simulink model "PFC"  (R2025a)
settings: Solver=VariableStepAuto  StartTime=0.0  StopTime=0.05  MaxStep=1e-9  RelTol=1e-3
libraries: spsDiodeLib x4, spsSeriesRLCBranchLib x2, spsACVoltageSourceLib x1, spsVoltageMeasurementLib x1, spspowerguiLib x1
settings Model: Creator=FCH  LastModifiedBy=FCH
settings DataIOCC: ReturnWorkspaceOutputs=off

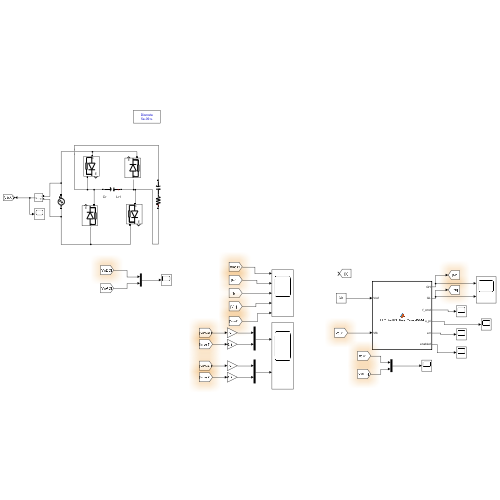
[thumbnail: Simulink's stored preview of the top-level diagram]
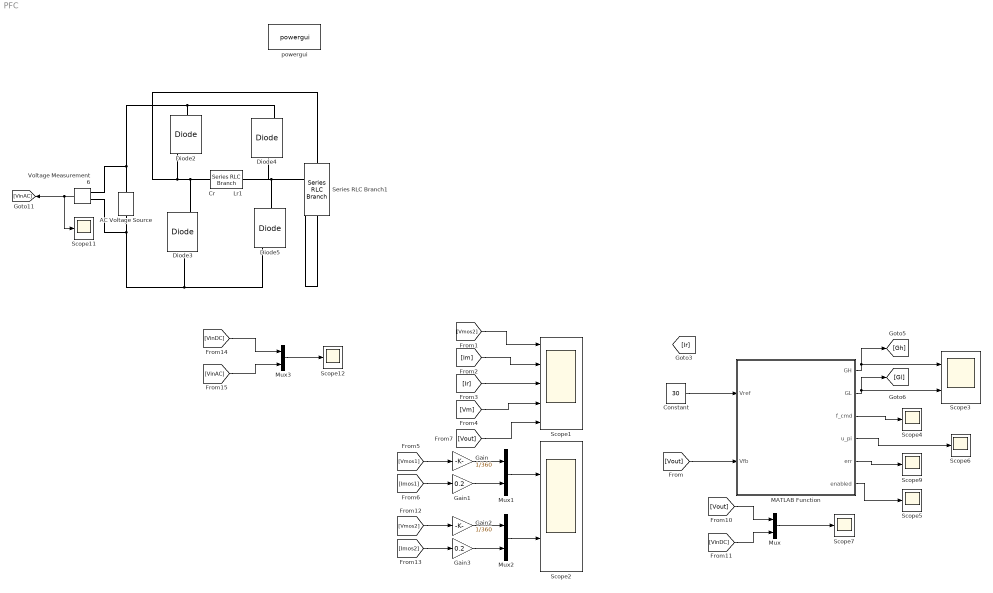
== system PFC ==
  AC Voltage Source : spsACVoltageSourceLib/AC Voltage Source  Amplitude=400  Phase=0  Frequency=50  SampleTime=0  Measurements=None  BusType=swing  Pref=10e3  Qref=0  Qmin=-inf  Qmax=+inf
  Constant : Constant  Value=30
  Cr           Lr1 : spsSeriesRLCBranchLib/Series RLC Branch  LConnTagsString=__new0  RConnTagsString=__new0  BranchType=C  Resistance=1000  Inductance=18e-6  SetiL0=off  InitialCurrent=0  Capacitance=1e-6  Setx0=off  InitialVoltage=0  Measurements=None
  Diode{2..5} (4 alike) : spsDiodeLib/Diode  Ron=0.001  Lon=0  Vf=0.8  IC=0  UseSnubber=0  Rs=500  Cs=250e-9  Measurements=on
  Gain : Gain  Gain=1/360
  Gain1 : Gain  Gain=0.2
  Gain2 : Gain  Gain=1/360
  Gain3 : Gain  Gain=0.2
  MATLAB Function : MATLAB Function  TreatAsAtomicUnit=on
  Mux{,1..3} (4 alike) : Mux  Inputs=2
  Scope1 : Scope  NumInputPorts=5
      settings: ActiveDisplayYMinimum=-50.08996079771358  ActiveDisplayYMaximum=450.08771732595056
  Scope{4..7,9,11..12} (7 alike) : Scope
      Scope11 settings: ActiveDisplayYMinimum=-499.86933273325383  ActiveDisplayYMaximum=498.82399459928456  DataLoggingVariableName=U_input1
      Scope12 settings: ActiveDisplayYMinimum=-62853.428585950089  ActiveDisplayYMaximum=-118.12720339930456  DataLoggingVariableName=ScopeData5
      Scope4 settings: ActiveDisplayYMinimum=222062.79129936235  ActiveDisplayYMaximum=225441.12510125362  DataLoggingVariableName=ScopeData4
      Scope5 settings: ActiveDisplayYMinimum=-0.12499999999999997  ActiveDisplayYMaximum=1.125  DataLoggingVariableName=ScopeData7
      Scope6 settings: ActiveDisplayYMinimum=-44.999999999999972  ActiveDisplayYMaximum=404.99999999999994  DataLoggingVariableName=ScopeData6
      Scope7 settings: ActiveDisplayYMinimum=-322.88834801894615  ActiveDisplayYMaximum=44.368039130053759  DataLoggingVariableName=ScopeData2
      Scope9 settings: ActiveDisplayYMinimum=-9.251113646286619  ActiveDisplayYMaximum=12.913805154194439  DataLoggingVariableName=ScopeData8
  Scope2 : Scope  NumInputPorts=2
      settings: ActiveDisplayYMinimum=-4.0516901529572973  ActiveDisplayYMaximum=20.70920117114095
  Scope3 : Scope  NumInputPorts=2
      settings: ActiveDisplayYMinimum=-0.12499999999999997  ActiveDisplayYMaximum=1.125  DataLoggingVariableName=ScopeData3
  Series RLC Branch1 : spsSeriesRLCBranchLib/Series RLC Branch  LConnTagsString=__new0  RConnTagsString=__new0  BranchType=RC  Resistance=0.01  Inductance=1e-3  SetiL0=off  InitialCurrent=0  Capacitance=1e-6  Setx0=off  InitialVoltage=0  Measurements=None
  Voltage Measurement6 : spsVoltageMeasurementLib/Voltage Measurement  PhasorSimulation=off  OutputType=Complex  PSBequivalent=0
  powergui : spspowerguiLib/powergui  Priority=1  SimulationMode=Discrete  SampleTime=1/(200e6)  frequency=60  Iterations=50  frequencyindice=0  Pbase=100e6  ErrMax=1e-4  UnitsV=kV  UnitsW=MW  buscounter=0  FunctionMessages=off  echomessages=off  EnableUseOfTLC=off  CurrentSourceSwitches=off  DisableSnubberDevices=off  DisableRonSwitches=off  DisableVfSwitches=off  DisplayEquations=off  AutomaticDiscreteSolvers=off  SolverType=Tustin/Backward Euler (TBE)  Interpol=off  ExternalGateDelay=off  methode=off  Ts=100  x0status=blocks  SPID=on  SwTol=0  HookPort=off  NonlinearTolerance=1e-4  nMaxIteration=100  ContinueOnMaxIteration=off  RestoreLinks=warning  ResistiveCurrentMeasurement=off  Frange=[0:2:500]  Ylog=off  Xlog=on  ShowGrid=off  save=off  variable=ZData  structure=0  ZoomFFT=off  StartTime=0.0  cycles=1  DisplayStyle=1  fundamental=60  FreqAxis=off  MaxFrequency=1000  frequencyindicesteady=1  RmsSteady=1  display=off
  wires:
  Constant/1 -> MATLAB Function/1(Vref)
  [Vout] -> MATLAB Function/2(Vfb)
  MATLAB Function/1(GH) -> [Gh], Scope3/1
  MATLAB Function/2(GL) -> [Gl], Scope3/2
  MATLAB Function/4(u_pi) -> Scope6/1
  MATLAB Function/3(f_cmd) -> Scope4/1
  MATLAB Function/5(err) -> Scope9/1
  [Vmos2] -> Scope1/1
  [Im] -> Scope1/2
  [Ir] -> Scope1/3
  [Vm] -> Scope1/4
  [Vout] -> Scope1/5
  Mux/1 -> Scope7/1
  [Vout] -> Mux/1
  [VinDC] -> Mux/2
  [Vmos1] -> Gain/1
  [Imos1] -> Gain1/1
  Mux1/1 -> Scope2/1
  [Vmos2] -> Gain2/1
  [Imos2] -> Gain3/1
  Mux2/1 -> Scope2/2
  Gain/1 -> Mux1/1
  Gain1/1 -> Mux1/2
  Gain2/1 -> Mux2/1
  Gain3/1 -> Mux2/2
  Voltage Measurement6/1 -> [VinAC], Scope11/1
  [VinDC] -> Mux3/1
  [VinAC] -> Mux3/2
  Mux3/1 -> Scope12/1
  MATLAB Function/6(enabled) -> Scope5/1
  connections:
  Cr           Lr1/LConn1 -- Diode4/LConn1 -- Series RLC Branch1/LConn1 -- Diode5/LConn1
  AC Voltage Source/RConn1 -- Diode4/RConn1 -- Diode2/LConn1 -- Voltage Measurement6/LConn2
  Diode5/RConn1 -- AC Voltage Source/LConn1 -- Voltage Measurement6/LConn1 -- Diode3/LConn1
  Diode2/RConn1 -- Series RLC Branch1/RConn1 -- Diode3/RConn1 -- Cr           Lr1/RConn1

== matlab function PFC/MATLAB Function ==
  data: Vref input; GH output; Vfb input; GL output; f_cmd output; u_pi output; err output; enabled output
function [GH, GL, f_cmd, u_pi, err, enabled] = LLC_VoltPI_Res_CompPWM(Vref, Vfb)
%#codegen
% LLC 变换器 PI 电压闭环 + 准谐振控制 + 互补 PWM 驱动（变频控制）
% 新增功能：准谐振控制消除9400Hz附近频率扰动
% 新增功能：0.02秒延时启动，0到0.02秒MOS管不导通
% 输入:
%   Vref  - 输出电压给定 (V)
%   Vfb   - 输出电压反馈 (V)
% 输出:
%   GH    - 高桥臂驱动（逻辑 0/1）
%   GL    - 低桥臂驱动（逻辑 0/1），与 GH 互补且带死区
%   f_cmd - 当前开关频率命令 (Hz)，便于观察
%   u_pi  - PI 控制器输出（归一化调节量，便于调试）
%   u_res - 准谐振控制器输出（便于调试）
%   u_total - 总控制输出（PI + 谐振）
%   err   - 误差值（便于调试）
%   enabled - 使能标志（0: 延时阶段，1: 正常运行）

% --- 控制周期（与 MATLAB Function 调用步长一致） ---
% Ts = 1/(270e3*20);          % 1 us 控制周期，例如 MCU 1 MHz ISR
Ts = 1/(2000e6);          % 0.5 ns 控制周期，用于高精度仿真
% Ts = 1/(1e6);             % 1 us 控制周期，MCU常见频率

% --- 启动延时参数 ---
startup_delay = 0.02/10;    % 启动延时 0.02 秒

% --- PI 参数（电压环）---
Kp = 0.00001;           % 比例系数
Ki = 50;                % 积分系数

% --- 准谐振控制器参数）---
Kr = 0.05;             % 谐振增益（需要根据实际调试）
f_res = 100;           % 谐振频率 (Hz) - 需要消除的扰动频率
omega_res = 2 * pi * f_res;  % 谐振角频率 (rad/s)

% 品质因数Q（影响带宽，Q越大带宽越窄，抑制越精确）
Q_res = 250000000;             % 品质因数

% --- LLC 开关频率范围 ---
f_min = 180e3;          % 最低频率 (Hz)
f_max = 270e3;          % 最高频率 (Hz)

% --- 死区时间 ---
t_dead = 186e-9;        % 200 ns 死区，根据驱动/器件调整

% --- 积分项限幅，防止积分饱和 ---
ui_max = 0.5;
ui_min = -0.5;

% --- 谐振控制器输出限幅 ---
u_res_max = 0.3;        % 谐振输出最大限幅
u_res_min = -0.3;       % 谐振输出最小限幅

% --- 总输出限幅 ---
u_total_max = 1.0;      % 总输出最大限幅
u_total_min = -1.0;     % 总输出最小限幅

%% ========= 持久变量（只初始化一次） =========
persistent ui t_half leg dead_t

% 准谐振控制器持久变量
persistent u_res_prev1 u_res_prev2  % 准谐振输出历史
persistent err_prev1 err_prev2      % 误差历史

% 离散化系数（只计算一次）
persistent b0_res b1_res b2_res a1_res a2_res

% 启动延时计时器
persistent startup_timer
persistent enable_flag

% 初始化
if isempty(ui)
    ui      = 0;        % PI 积分项
    t_half  = 0;        % 半周期计时
    leg     = int8(0);  % 当前导通臂：0=上臂导通，1=下臂导通
    dead_t  = 0;        % 当前死区计时
    
    % 准谐振控制器初始化
    u_res_prev1 = 0;    % 前一次谐振输出
    u_res_prev2 = 0;    % 前两次谐振输出
    err_prev1 = 0;      % 前一次误差
    err_prev2 = 0;      % 前两次误差
    
    % 启动延时初始化
    startup_timer = 0;
    enable_flag = false;
    
    % 计算准谐振控制器离散化系数（使用双线性变换）
    % 连续传递函数: H(s) = Kr * (omega_res/Q_res) * s / (s^2 + (omega_res/Q_res)*s + omega_res^2)
    
    T = Ts;
    w0 = omega_res;
    Kr_gain = Kr;
    Q = Q_res;
    
    % 预扭曲处理以保持谐振频率准确
    w0_prewarp = (2/T) * tan(w0 * T/2);
    
    % 双线性变换: s = (2/T) * (z-1)/(z+1)
    % 计算离散系数
    den = (w0_prewarp/Q)^2 + w0_prewarp^2 + 4/T^2 + 4*w0_prewarp/(Q*T);
    
    b0_res = (4*Kr_gain*w0_prewarp/(Q*T)) / den;
    b1_res = 0;
    b2_res = -b0_res;
    a1_res = (2*w0_prewarp^2 - 8/T^2) / den;
    a2_res = (4/T^2 - 4*w0_prewarp/(Q*T) + (w0_prewarp/Q)^2 + w0_prewarp^2) / den;
end

%% ========= 启动延时逻辑 =========
% 更新启动计时器
startup_timer = startup_timer + Ts;

% 检查是否达到启动延时时间
if startup_timer >= startup_delay
    enable_flag = true;
end

% 设置输出使能标志
if enable_flag
    enabled = true;
else
    enabled = false;
end

%% ========= 0-0.02秒：延时启动阶段 =========
if ~enable_flag
    % 在启动延时期间，MOS管不导通
    GH = false;
    GL = false;
    
    % 其他输出设置为0或默认值
    f_cmd = 0;
    u_pi = 0;
    u_res = 0;
    u_total = 0;
    err = 0;
    
    % 在延时阶段，可以初始化一些变量，但不更新控制状态
    % 这里可以选择更新误差历史，或者保持为0
    
    return;  % 直接返回，不执行后续的控制逻辑
end

%% ========= 1. 电压误差 & PI 电压环 =========
err = Vref - Vfb;      % 电压误差：Vref - Vfb

% 比例项
up = Kp * err;

% 积分项更新（带抗饱和）
ui_new = ui + Ki * Ts * err;

% 积分限幅
if ui_new > ui_max
    ui_new = ui_max;
elseif ui_new < ui_min
    ui_new = ui_min;
end
ui = ui_new;

% PI 输出
u_pi = up + ui;

%% ========= 2. 准谐振控制器（消除9400Hz扰动） =========
% 方法1：直接IIR滤波器实现（更稳定）
u_res = b0_res * err + b1_res * err_prev1 + b2_res * err_prev2 ...
        - a1_res * u_res_prev1 - a2_res * u_res_prev2;

% 谐振输出限幅
if u_res > u_res_max
    u_res = u_res_max;
elseif u_res < u_res_min
    u_res = u_res_min;
end

% 更新历史状态
err_prev2 = err_prev1;
err_prev1 = err;
u_res_prev2 = u_res_prev1;
u_res_prev1 = u_res;

%% ========= 3. 总控制输出 =========
u_total = u_pi + u_res;

% 总输出限幅
if u_total > u_total_max
    u_total = u_total_max;
elseif u_total < u_total_min
    u_total = u_total_min;
end

%% ========= 4. 总控制输出映射为开关频率命令 =========
% u_total 在 [-1, 1] 范围内映射到频率范围 [f_min, f_max]
u_norm = 0.5 + 0.5 * u_total;  % 映射到 [0, 1]

% 保证在 [0,1] 内
if u_norm > 1
    u_norm = 1;
elseif u_norm < 0
    u_norm = 0;
end

% 映射到频率范围 [f_min, f_max]
f_cmd = f_min + u_norm * (f_max - f_min);

% 频率限幅
if f_cmd > f_max
    f_cmd = f_max;
elseif f_cmd < f_min
    f_cmd = f_min;
end

%% ========= 5. 根据频率命令生成 50% 占空方波 =========
% 半周期 = 1 / (2 * f_cmd)
T_half = 1.0 / (2.0 * f_cmd);

% 半周期计数
t_half = t_half + Ts;

% 每经过一个半周期翻转一次桥臂导通状态
if t_half >= T_half
    t_half = t_half - T_half;     % 保持时间误差不积累
    leg    = bitxor(leg, int8(1));% 0 <-> 1 翻转导通臂
    dead_t = t_dead;              % 每次换向都重新启动死区
end

%% ========= 6. 互补 PWM + 死区逻辑 =========
% 在死区时间内，两臂都关闭
if dead_t > 0
    dead_t = dead_t - Ts;
    GH = false;
    GL = false;
else
    % 死区结束后，根据 leg 状态驱动互补 PWM
    if leg == 0
        GH = true;     % 上臂导通
        GL = false;    % 下臂关闭
    else
        GH = false;    % 上臂关闭
        GL = true;     % 下臂导通
    end
end

end
